simulink model "cruise_control"  (R2018a)
settings: Solver=VariableStepAuto  StartTime=0.0  StopTime=10.0  RelTol=1e-3
PreLoadFcn:
  | load('cruise_control.mat')
values from neighbouring files (symbols this model uses):
  Ki = 1    [cruise_control.mat]
  Kp = 1    [cruise_control.mat]
settings Model: Creator=rl185160  LastModifiedBy=rl185160

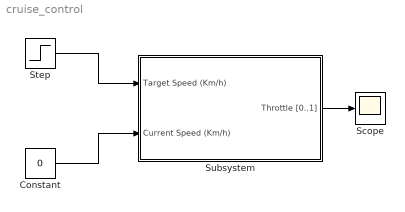
== system cruise_control ==
  "Constant " : Constant  Value=0
  Scope : Scope
  "Step " : Step  After=0.1  SampleTime=0
  Subsystem : Subsystem
  wires:
  "Step "/1 -> Subsystem/1(Target Speed (Km/h))
  "Constant "/1 -> Subsystem/2(Current Speed (Km/h))
  Subsystem/1(Throttle [0..1]) -> Scope/1

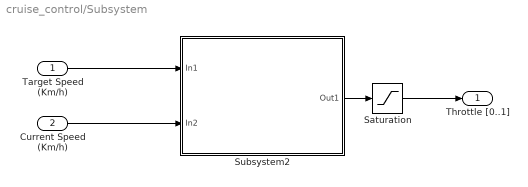
== system cruise_control/Subsystem ==
  Target Speed (Km/h) : Inport
  Current Speed (Km/h) : Inport  Port=2
  Saturation : Saturate  UpperLimit=1  LowerLimit=0
  Subsystem2 : Subsystem
  Throttle [0..1] : Outport
  wires:
  Saturation/1 -> Throttle [0..1]/1
  Target Speed (Km/h)/1 -> Subsystem2/1(In1)
  Current Speed (Km/h)/1 -> Subsystem2/2(In2)
  Subsystem2/1(Out1) -> Saturation/1

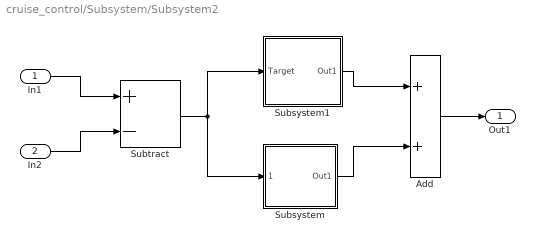
== system cruise_control/Subsystem/Subsystem2 ==
  In1 : Inport
  In2 : Inport  Port=2
  Add : Sum
  Subsystem : Subsystem
  Subsystem1 : Subsystem
  Subtract : Sum  Inputs=+-
  Out1 : Outport
  wires:
  In1/1 -> Subtract/1
  Subsystem/1(Out1) -> Add/2
  Add/1 -> Out1/1
  In2/1 -> Subtract/2
  Subsystem1/1(Out1) -> Add/1
  Subtract/1 -> Subsystem1/1("Target "), Subsystem/1(" ")

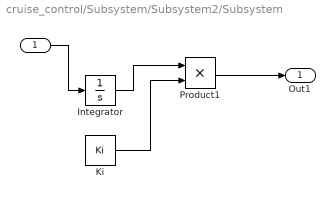
== system cruise_control/Subsystem/Subsystem2/Subsystem ==
  " " : Inport
  Integrator : Integrator
  "Ki " : Constant  Value=Ki
  Product1 : Product
  Out1 : Outport
  wires:
  Product1/1 -> Out1/1
  "Ki "/1 -> Product1/2
  " "/1 -> Integrator/1
  Integrator/1 -> Product1/1

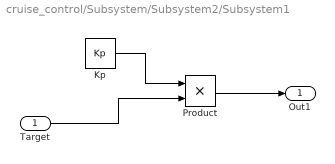
== system cruise_control/Subsystem/Subsystem2/Subsystem1 ==
  "Target " : Inport
  "Kp " : Constant  Value=Kp
  Product : Product
  Out1 : Outport
  wires:
  Product/1 -> Out1/1
  "Target "/1 -> Product/2
  "Kp "/1 -> Product/1
